simulink model "EcatHandler"  (R2016b)
settings: Solver=FixedStepDiscrete  StartTime=0.0  StopTime=inf  FixedStep=0.002  RelTol=1e-3  EnableMultiTasking=on
libraries: xpcethercatlib x22
settings Model: xpc_rtwmakecfg_data=_xpcethercatlib_  Creator=march  LastModifiedBy=march
settings SolverCC: EnableConcurrentExecution=on  AutoInsertRateTranBlk=on
settings DataIOCC: SaveFormat=StructureWithTime  SaveOutput=off  SaveTime=off
settings OptimizationCC: BlockReduction=off  OptimizeBlockIOStorage=off  BufferReuse=off  GlobalBufferReuse=off  ExpressionFolding=off  LocalBlockOutputs=off
settings HardwareCC: ProdBitPerPointer=32  ProdBitPerSizeT=32  ProdBitPerPtrDiffT=32  ProdLargestAtomicFloat=None  ProdWordSize=32  ProdLongLongMode=on  ProdHWDeviceType=Generic->32-bit x86 compatible
settings ModelReferenceCC: ModelReferenceNumInstancesAllowed=Single
settings RTWCC: SystemTargetFile=slrt.tlc  TemplateMakefile=slrt_default_tmf  PostCodeGenCommand=SomanetTuning_make_rtw_hook  Description=Simulink Real-Time  RTWVerbose=off  CodeExecutionProfiling=on  RTWCompilerOptimization=on
settings SimulinkRealTimeCC: xPCModelTimeoutSecs=20

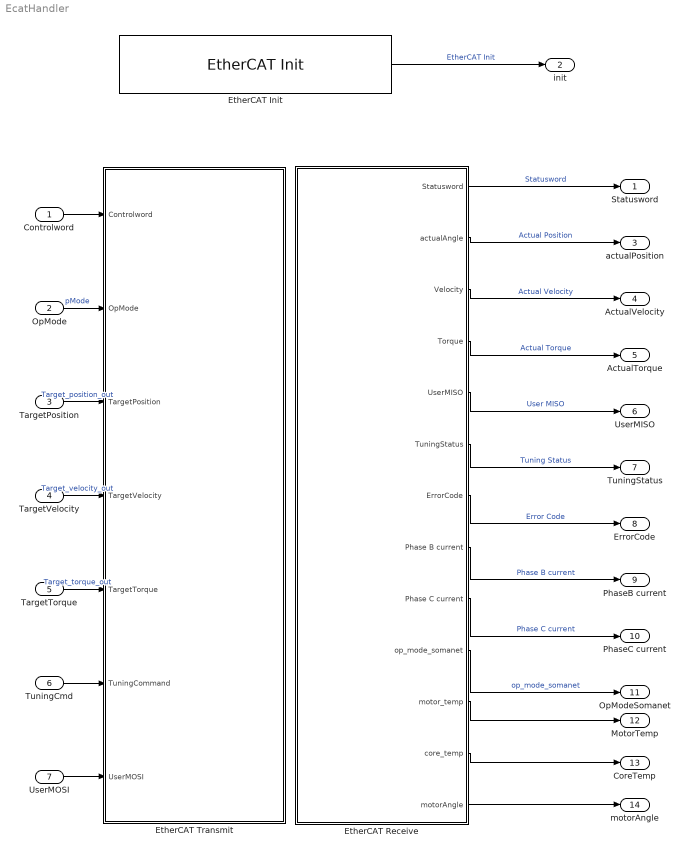
== system EcatHandler ==
  Controlword : Inport  OutDataTypeStr=uint16  PortDimensions=1  SampleTime=[0.002,0]
  OpMode : Inport  Port=2  OutDataTypeStr=int8  PortDimensions=1  SampleTime=[0.002,0]
  TargetPosition : Inport  Port=3  OutDataTypeStr=int32  PortDimensions=1  SampleTime=[0.002,0]
  TargetVelocity : Inport  Port=4  OutDataTypeStr=int32  PortDimensions=1  SampleTime=[0.002,0]
  TargetTorque : Inport  Port=5  OutDataTypeStr=int16  PortDimensions=1  SampleTime=[0.002,0]
  TuningCmd : Inport  Port=6  OutDataTypeStr=uint32  PortDimensions=1  SampleTime=[0.002,0]
  UserMOSI : Inport  Port=7  OutDataTypeStr=uint32  PortDimensions=1  SampleTime=[0.002,0]
  "EtherCAT Init " : xpcethercatlib/EtherCAT Init   Priority=0  config_file=D:\Software\Team_16-17\simulink-models\EcatXML\SingleJoint_eni.xml  device_id=0  pci_bus=2  pci_slot=0  dctuning=0  enaDebug=off  enaDC=on  errLink=off  masterDbg=off  stateChgDbg=off  baseClock=off  masterCfg=off  logFile='c:\dbglog.txt'  sample_time=0.002000  DCMode=0
  EtherCAT Receive : Subsystem
  EtherCAT Transmit : Subsystem
  Statusword : Outport  OutDataTypeStr=uint16  PortDimensions=1  SampleTime=[0.002,0]
  init : Outport  Port=2  OutDataTypeStr=int32  PortDimensions=6  SampleTime=[0.002,0]
  actualPosition : Outport  Port=3  OutDataTypeStr=int32  PortDimensions=1  SampleTime=[0.002,0]
  ActualVelocity : Outport  Port=4  OutDataTypeStr=int32  PortDimensions=1  SampleTime=[0.002,0]
  ActualTorque : Outport  Port=5  OutDataTypeStr=int16  PortDimensions=1  SampleTime=[0.002,0]
  UserMISO : Outport  Port=6  OutDataTypeStr=uint32  PortDimensions=1  SampleTime=[0.002,0]
  TuningStatus : Outport  Port=7  OutDataTypeStr=uint32  PortDimensions=1  SampleTime=[0.002,0]
  ErrorCode : Outport  Port=8  OutDataTypeStr=double  PortDimensions=1  SampleTime=[0.002,0]
  PhaseB current : Outport  Port=9  OutDataTypeStr=int16  PortDimensions=1  SampleTime=[0.002,0]
  PhaseC current : Outport  Port=10  OutDataTypeStr=int16  PortDimensions=1  SampleTime=[0.002,0]
  OpModeSomanet : Outport  Port=11  OutDataTypeStr=int8  PortDimensions=1  SampleTime=[0.002,0]
  MotorTemp : Outport  Port=12  OutDataTypeStr=single  PortDimensions=1  SampleTime=[0.002,0]
  CoreTemp : Outport  Port=13  OutDataTypeStr=int16  PortDimensions=1  SampleTime=[0.002,0]
  motorAngle : Outport  Port=14  OutDataTypeStr=int32  PortDimensions=1  SampleTime=[0.002,0]
  wires:
  OpMode/1 -> EtherCAT Transmit/2(OpMode)  "pMode"
  EtherCAT Receive/11(motor_temp) -> MotorTemp/1
  EtherCAT Receive/12(core_temp) -> CoreTemp/1
  UserMOSI/1 -> EtherCAT Transmit/7(UserMOSI)
  EtherCAT Receive/7(ErrorCode) -> ErrorCode/1  "Error Code"
  EtherCAT Receive/5(UserMISO) -> UserMISO/1  "User MISO"
  Controlword/1 -> EtherCAT Transmit/1("Controlword ")
  TuningCmd/1 -> EtherCAT Transmit/6(TuningCommand)
  EtherCAT Receive/6(TuningStatus) -> TuningStatus/1  "Tuning Status"
  TargetTorque/1 -> EtherCAT Transmit/5(TargetTorque)  "Target_torque_out"
  TargetVelocity/1 -> EtherCAT Transmit/4(TargetVelocity)  "Target_velocity_out"
  TargetPosition/1 -> EtherCAT Transmit/3(TargetPosition)  "Target_position_out"
  EtherCAT Receive/1(Statusword) -> Statusword/1  "Statusword"
  EtherCAT Receive/2(actualAngle) -> actualPosition/1  "Actual Position"
  EtherCAT Receive/3(Velocity) -> ActualVelocity/1  "Actual Velocity"
  EtherCAT Receive/4(Torque) -> ActualTorque/1  "Actual Torque"
  EtherCAT Receive/9(Phase C current) -> PhaseC current/1  "Phase C current"
  EtherCAT Receive/8(Phase B current) -> PhaseB current/1  "Phase B current"
  EtherCAT Receive/10(op_mode_somanet) -> OpModeSomanet/1  "op_mode_somanet"
  "EtherCAT Init "/1 -> init/1  "EtherCAT Init"
  EtherCAT Receive/13(motorAngle) -> motorAngle/1

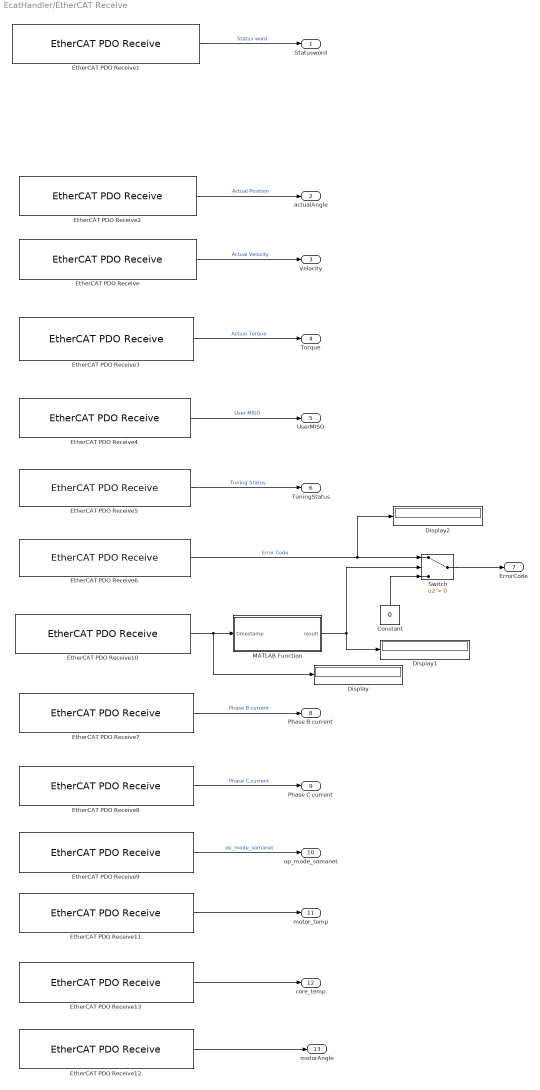
== system EcatHandler/EtherCAT Receive ==
  Constant : Constant  Value=0
  Display : Display
  Display1 : Display
  Display2 : Display
  EtherCAT PDO Receive : xpcethercatlib/EtherCAT PDO Receive  Priority=2  sig_name=Drive 1 (CiA402 Motor Control Device).Inputs.Velocity Value  sig_offset=264  sig_type=int32  type_size=32  sig_dim=1  device_id=0  sample_time=0.002000
  EtherCAT PDO Receive1 : xpcethercatlib/EtherCAT PDO Receive  Priority=2  sig_name=Drive 1 (CiA402 Motor Control Device).Inputs.Statusword  sig_offset=208  sig_type=uint16  type_size=16  sig_dim=1  device_id=0  sample_time=0.002000
  EtherCAT PDO Receive10 : xpcethercatlib/EtherCAT PDO Receive  Priority=2  sig_name=Drive 1 (CiA402 Motor Control Device).Inputs.timestamp  sig_offset=536  sig_type=uint32  type_size=32  sig_dim=1  device_id=0  sample_time=0.002000
  EtherCAT PDO Receive11 : xpcethercatlib/EtherCAT PDO Receive  Priority=2  sig_name=Box 2 (EasyCAT 32+32 configurable PDO).Inputs.temperature  sig_offset=728  sig_type=single  type_size=32  sig_dim=1  device_id=0  sample_time=0.002000
  EtherCAT PDO Receive12 : xpcethercatlib/EtherCAT PDO Receive  Priority=2  sig_name=Drive 1 (CiA402 Motor Control Device).Inputs.Secondary position value  sig_offset=312  sig_type=int32  type_size=32  sig_dim=1  device_id=0  sample_time=0.002000
  EtherCAT PDO Receive13 : xpcethercatlib/EtherCAT PDO Receive  Priority=2  sig_name=Drive 1 (CiA402 Motor Control Device).Inputs.Core Temp  sig_offset=616  sig_type=int16  type_size=16  sig_dim=1  device_id=0  sample_time=0.002000
  EtherCAT PDO Receive2 : xpcethercatlib/EtherCAT PDO Receive  Priority=2  sig_name=Drive 1 (CiA402 Motor Control Device).Inputs.Position Value  sig_offset=232  sig_type=int32  type_size=32  sig_dim=1  device_id=0  sample_time=0.002000
  EtherCAT PDO Receive3 : xpcethercatlib/EtherCAT PDO Receive  Priority=2  sig_name=Drive 1 (CiA402 Motor Control Device).Inputs.Torque Value  sig_offset=296  sig_type=int16  type_size=16  sig_dim=1  device_id=0  sample_time=0.002000
  EtherCAT PDO Receive4 : xpcethercatlib/EtherCAT PDO Receive  Priority=2  sig_name=Drive 1 (CiA402 Motor Control Device).Inputs.User MISO  sig_offset=504  sig_type=uint32  type_size=32  sig_dim=1  device_id=0  sample_time=0.002000
  EtherCAT PDO Receive5 : xpcethercatlib/EtherCAT PDO Receive  Priority=2  sig_name=Drive 1 (CiA402 Motor Control Device).Inputs.Tuning status  sig_offset=440  sig_type=uint32  type_size=32  sig_dim=1  device_id=0  sample_time=0.002000
  EtherCAT PDO Receive6 : xpcethercatlib/EtherCAT PDO Receive  Priority=2  sig_name=Drive 1 (CiA402 Motor Control Device).Inputs.Error code  sig_offset=568  sig_type=uint16  type_size=16  sig_dim=1  device_id=0  sample_time=0.002000
  EtherCAT PDO Receive7 : xpcethercatlib/EtherCAT PDO Receive  Priority=2  sig_name=Drive 1 (CiA402 Motor Control Device).Inputs.Phase B  sig_offset=584  sig_type=int16  type_size=16  sig_dim=1  device_id=0  sample_time=0.002000
  EtherCAT PDO Receive8 : xpcethercatlib/EtherCAT PDO Receive  Priority=2  sig_name=Drive 1 (CiA402 Motor Control Device).Inputs.Phase C  sig_offset=600  sig_type=int16  type_size=16  sig_dim=1  device_id=0  sample_time=0.002000
  EtherCAT PDO Receive9 : xpcethercatlib/EtherCAT PDO Receive  Priority=2  sig_name=Drive 1 (CiA402 Motor Control Device).Inputs.Op Mode Display  sig_offset=224  sig_type=int8  type_size=8  sig_dim=1  device_id=0  sample_time=0.002000
  MATLAB Function : MATLAB Function  TreatAsAtomicUnit=on
  Switch : Switch  Criteria=u2 > Threshold
  Statusword : Outport
  actualAngle : Outport  Port=2
  Velocity : Outport  Port=3
  Torque : Outport  Port=4
  UserMISO : Outport  Port=5
  TuningStatus : Outport  Port=6
  ErrorCode : Outport  Port=7
  Phase B current : Outport  Port=8
  Phase C current : Outport  Port=9
  op_mode_somanet : Outport  Port=10
  motor_temp : Outport  Port=11
  core_temp : Outport  Port=12
  motorAngle : Outport  Port=13
  wires:
  EtherCAT PDO Receive11/1 -> motor_temp/1
  EtherCAT PDO Receive13/1 -> core_temp/1
  Constant/1 -> Switch/3
  MATLAB Function/1(result) -> Display1/1, Switch/2
  Switch/1 -> ErrorCode/1
  EtherCAT PDO Receive10/1 -> MATLAB Function/1(timestamp), Display/1
  EtherCAT PDO Receive9/1 -> op_mode_somanet/1  "op_mode_somanet"
  EtherCAT PDO Receive8/1 -> Phase C current/1  "Phase C current"
  EtherCAT PDO Receive7/1 -> Phase B current/1  "Phase B current"
  EtherCAT PDO Receive6/1 -> Switch/1, Display2/1  "Error Code"
  EtherCAT PDO Receive5/1 -> TuningStatus/1  "Tuning Status"
  EtherCAT PDO Receive4/1 -> UserMISO/1  "User MISO"
  EtherCAT PDO Receive3/1 -> Torque/1  "Actual Torque"
  EtherCAT PDO Receive2/1 -> actualAngle/1  "Actual Position"
  EtherCAT PDO Receive/1 -> Velocity/1  "Actual Velocity"
  EtherCAT PDO Receive1/1 -> Statusword/1  "Status word"
  EtherCAT PDO Receive12/1 -> motorAngle/1

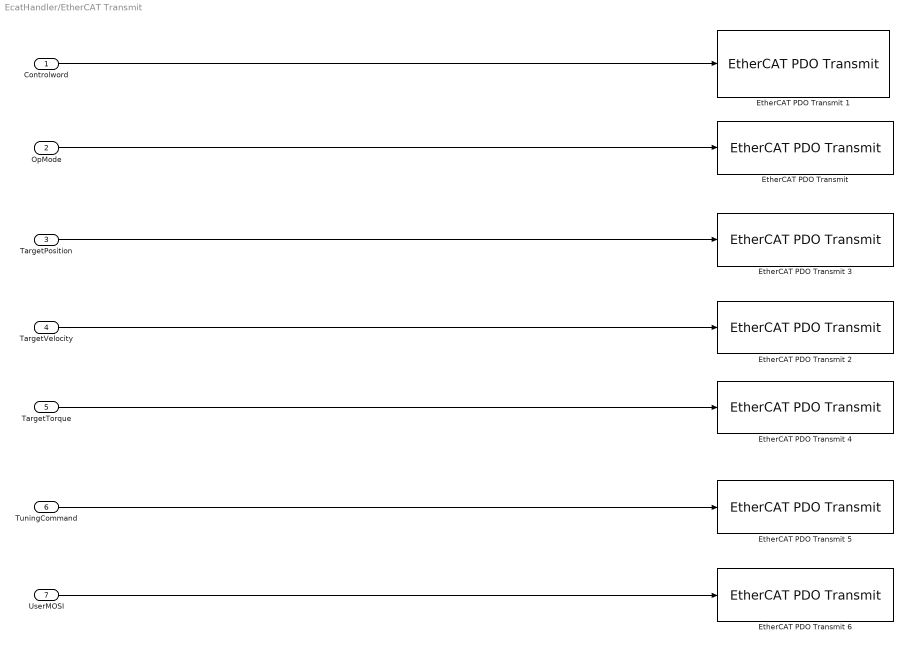
== system EcatHandler/EtherCAT Transmit ==
  "Controlword " : Inport
  OpMode : Inport  Port=2
  TargetPosition : Inport  Port=3
  TargetVelocity : Inport  Port=4
  TargetTorque : Inport  Port=5
  TuningCommand : Inport  Port=6
  UserMOSI : Inport  Port=7
  "EtherCAT PDO Transmit " : xpcethercatlib/EtherCAT PDO Transmit   Priority=3  sig_name=Drive 1 (CiA402 Motor Control Device).Outputs.Op Mode  sig_offset=224  sig_type=int8  type_size=8  sig_dim=1  device_id=0  sample_time=0.002000
  EtherCAT PDO Transmit 1 : xpcethercatlib/EtherCAT PDO Transmit   Priority=3  sig_name=Drive 1 (CiA402 Motor Control Device).Outputs.Controlword  sig_offset=208  sig_type=uint16  type_size=16  sig_dim=1  device_id=0  sample_time=0.002000
  EtherCAT PDO Transmit 2 : xpcethercatlib/EtherCAT PDO Transmit   Priority=3  sig_name=Drive 1 (CiA402 Motor Control Device).Outputs.Target Velocity  sig_offset=280  sig_type=int32  type_size=32  sig_dim=1  device_id=0  sample_time=0.002000
  EtherCAT PDO Transmit 3 : xpcethercatlib/EtherCAT PDO Transmit   Priority=3  sig_name=Drive 1 (CiA402 Motor Control Device).Outputs.Target Position  sig_offset=248  sig_type=int32  type_size=32  sig_dim=1  device_id=0  sample_time=0.002000
  EtherCAT PDO Transmit 4 : xpcethercatlib/EtherCAT PDO Transmit   Priority=3  sig_name=Drive 1 (CiA402 Motor Control Device).Outputs.Target Torque  sig_offset=232  sig_type=int16  type_size=16  sig_dim=1  device_id=0  sample_time=0.002000
  EtherCAT PDO Transmit 5 : xpcethercatlib/EtherCAT PDO Transmit   Priority=3  sig_name=Drive 1 (CiA402 Motor Control Device).Outputs.Tuning command  sig_offset=344  sig_type=uint32  type_size=32  sig_dim=1  device_id=0  sample_time=0.002000
  EtherCAT PDO Transmit 6 : xpcethercatlib/EtherCAT PDO Transmit   Priority=3  sig_name=Drive 1 (CiA402 Motor Control Device).Outputs.User MOSI  sig_offset=408  sig_type=uint32  type_size=32  sig_dim=1  device_id=0  sample_time=0.002000
  wires:
  UserMOSI/1 -> EtherCAT PDO Transmit 6/1
  TuningCommand/1 -> EtherCAT PDO Transmit 5/1
  TargetTorque/1 -> EtherCAT PDO Transmit 4/1
  TargetPosition/1 -> EtherCAT PDO Transmit 3/1
  OpMode/1 -> "EtherCAT PDO Transmit "/1
  "Controlword "/1 -> EtherCAT PDO Transmit 1/1
  TargetVelocity/1 -> EtherCAT PDO Transmit 2/1

== matlab function EcatHandler/EtherCAT Receive/MATLAB Function ==
  data: timestamp input; result output
function result = isconnected(timestamp)
persistent timestamps;
persistent entry;

if(isempty(timestamps))
    timestamps = uint32((1:2500)');
    entry = 1;
end

timestamps(entry) = timestamp;
entry = mod(entry,2500);
entry = entry + 1;
if min(timestamps)~=max(timestamps)
    % now the somanet is connected, so we give a result ~= 0 
    % this means the actual error code gets sent
    result = 1;
else
    % now errorcode=0
    result = 0;
end
%result = 1;
end
